simulink model "files_continuous_write_test"  (R2022a)
settings: Solver=FixedStepDiscrete  StartTime=0.0  StopTime=inf  FixedStep=0.001  MaxStep=0.001  RelTol=1e-3
undefined symbols (not defined in the file): CR, LF
libraries: dspstat3 x4, simulink x3, instrumentlib x2, matrix_library x1, slrealtimeutilitieslib x1, commcrc2 x1
settings Model: SimulationMode=accelerator  Creator=DeveloperY  LastModifiedBy=DeveloperY
settings SolverCC: AllowMultiTaskInputOutput=on  ConcurrentTasks=on

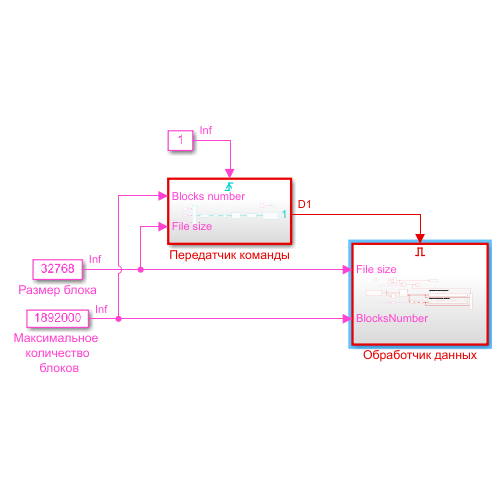
[thumbnail: Simulink's stored preview of the top-level diagram]
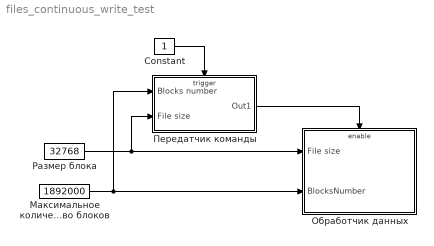
== system files_continuous_write_test ==
  Constant : Constant
  Максимальное количество блоков : Constant  Value=1892000  OutDataTypeStr=uint32
  Обработчик данных : Subsystem  TreatAsAtomicUnit=on
  Передатчик команды : Subsystem  TreatAsAtomicUnit=on
  Размер блока : Constant  Value=32768  OutDataTypeStr=uint32
  wires:
  Constant/1 -> Передатчик команды/Trigger
  Максимальное количество блоков/1 -> Передатчик команды/1(Blocks number), Обработчик данных/2(BlocksNumber)
  Размер блока/1 -> Обработчик данных/1(File size), Передатчик команды/2(File size)
  Передатчик команды/1(Out1) -> Обработчик данных/Enable

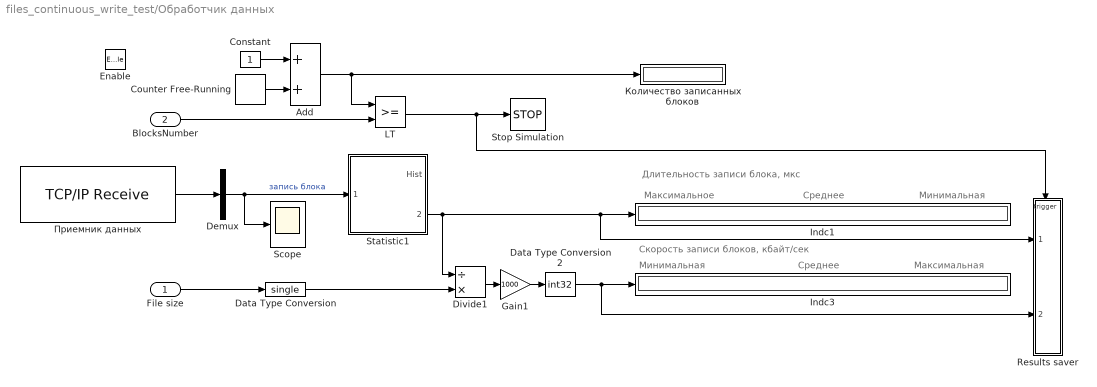
== system files_continuous_write_test/Обработчик данных ==
  note: Длительность записи блока, мкс
  note: Минимальная
  note: Среднее
  note: Максимальное
  note: Максимальная
  note: Среднее
  note: Минимальная
  note: Скорость записи блоков, кбайт/сек
  File size : Inport
  BlocksNumber : Inport  Port=2
  Enable : EnablePort
  " Indc1" : Display
  Add : Sum
  Constant : Constant
  Counter Free-Running : simulink/Sources/Counter Free-Running  NumBits=32  tsamp=-1
  Data Type Conversion : DataTypeConversion  OutDataTypeStr=single  SaturateOnIntegerOverflow=off  RndMeth=Floor
  Data Type Conversion2 : DataTypeConversion  OutDataTypeStr=int32  SaturateOnIntegerOverflow=off  RndMeth=Floor
  Demux : Demux  Outputs=1
  Divide1 : Product  Inputs=/*  OutDataTypeStr=single
  Gain1 : Gain  Gain=1000
  Indc3 : Display
  LT : RelationalOperator  OutDataTypeStr=boolean  RndMeth=Simplest  InputSameDT=off
  Results saver : Subsystem  TreatAsAtomicUnit=on
  Scope : Scope
  Statistic1 : Subsystem
  Stop Simulation : Stop
  Количество записанных блоков : Display
  Приемник данных : instrumentlib/TCP//IP Receive  Host=192.168.3.1  Port=3333  DataSize=[1]  DataType=ASCII  ASCIIFormatting=%d  Terminator=CR/LF  CustomTerminator=10  ByteOrder=big-endian  EnableBlockingMode=on  Timeout=10  SampleTime=-1  SimulateUsing=Interpreted execution
  wires:
  Demux/1 -> Scope/1, Statistic1/1(Samples)  "запись блока"
  Add/1 -> LT/1, Количество записанных блоков/1
  Statistic1/2(Duration) -> Divide1/1, " Indc1"/1, Results saver/1(Duration)
  File size/1 -> Data Type Conversion/1
  LT/1 -> Stop Simulation/1, Results saver/Trigger
  Data Type Conversion/1 -> Divide1/2
  Gain1/1 -> Data Type Conversion2/1
  Data Type Conversion2/1 -> Results saver/2(Speed), Indc3/1
  Divide1/1 -> Gain1/1
  BlocksNumber/1 -> LT/2
  Counter Free-Running/1 -> Add/2
  Constant/1 -> Add/1
  Приемник данных/1 -> Demux/1

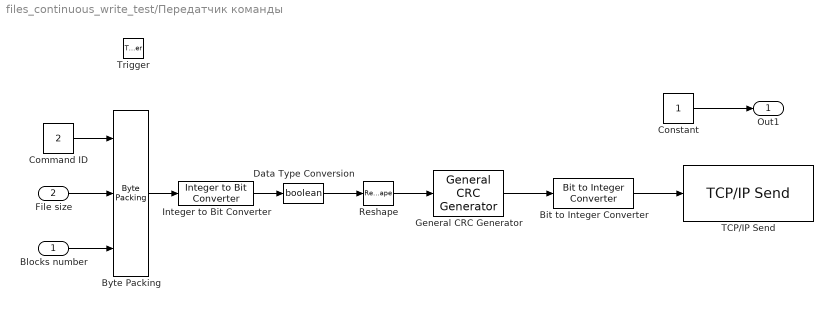
== system files_continuous_write_test/Передатчик команды ==
  Blocks number : Inport
  File size : Inport  Port=2
  Trigger : TriggerPort  VariantControl=(inherit)  InitialTriggerSignalState=zero
  Bit to Integer Converter : simulink/Logic and Bit Operations/Bit to Integer Converter  nbits=8  bitOrder=MSB first  signedOutputValues=Unsigned  outDtype=Inherit via internal rule  outDtypeSigned=Inherit via internal rule
      settings: SourceProductBaseCode=SL
  Byte Packing : slrealtimeutilitieslib/Byte Packing  MaskPackedDataType=uint8  MaskUnpackedDataTypes={'uint32','uint32','uint32' }  MaskAlignment=1
  Command ID : Constant  Value=2  OutDataTypeStr=uint32
  Constant : Constant
  Data Type Conversion : DataTypeConversion  OutDataTypeStr=boolean  SaturateOnIntegerOverflow=off  RndMeth=Floor
  General CRC Generator : commcrc2/General CRC Generator  genPoly='z^16 + z^12 + z^5 + 1'  iniStates=0  directMethod=off  reflectInputBytes=off  reflectChecksums=off  finalXOR=0  numChecksums=1
      settings: SourceProductBaseCode=CM
  Integer to Bit Converter : simulink/Logic and Bit Operations/Integer to Bit Converter  nbits=8  signedInputValues=Unsigned  bitOrder=MSB first  outDtype=Inherit via internal rule
      settings: SourceProductBaseCode=SL
  Reshape : Reshape  OutputDimensionality=Customize  OutputDimensions=[96,1]
  TCP/IP Send : instrumentlib/TCP//IP Send  Host=192.168.3.1  Port=3333  ByteOrder=big-endian  EnableBlockingMode=off  Timeout=0.1  TransferDelay=on  SimulateUsing=Interpreted execution
  Out1 : Outport
  wires:
  Command ID/1 -> Byte Packing/1
  File size/1 -> Byte Packing/2
  Blocks number/1 -> Byte Packing/3
  Integer to Bit Converter/1 -> Data Type Conversion/1
  Data Type Conversion/1 -> Reshape/1
  Reshape/1 -> General CRC Generator/1
  General CRC Generator/1 -> Bit to Integer Converter/1
  Bit to Integer Converter/1 -> TCP/IP Send/1
  Byte Packing/1 -> Integer to Bit Converter/1
  Constant/1 -> Out1/1

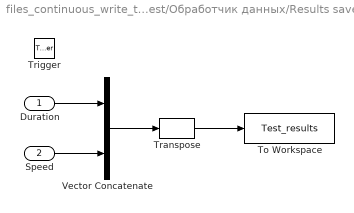
== system files_continuous_write_test/Обработчик данных/Results saver ==
  Duration : Inport
  Speed : Inport  Port=2
  Trigger : TriggerPort  VariantControl=(inherit)  InitialTriggerSignalState=zero
  To Workspace : ToWorkspace  VariableName=Test_results  SampleTime=-1
  Transpose : matrix_library/Transpose
      settings: SourceProductBaseCode=SL
  Vector Concatenate : Concatenate  Mode=Multidimensional array  ConcatenateDimension=2
  wires:
  Duration/1 -> Vector Concatenate/1
  Vector Concatenate/1 -> Transpose/1
  Transpose/1 -> To Workspace/1
  Speed/1 -> Vector Concatenate/2

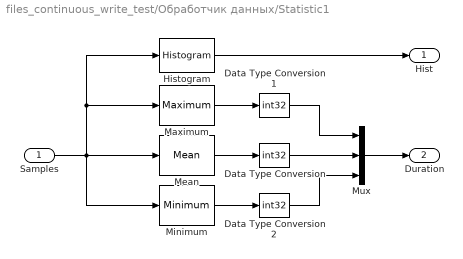
== system files_continuous_write_test/Обработчик данных/Statistic1 ==
  Samples : Inport
  Data Type Conversion : DataTypeConversion  OutDataTypeStr=int32  SaturateOnIntegerOverflow=off  RndMeth=Floor
  Data Type Conversion1 : DataTypeConversion  OutDataTypeStr=int32  SaturateOnIntegerOverflow=off  RndMeth=Floor
  Data Type Conversion2 : DataTypeConversion  OutDataTypeStr=int32  SaturateOnIntegerOverflow=off  RndMeth=Floor
  Histogram : dspstat3/Histogram  umin=0  umax=1000000  nbins=100  operateOver=Entire input  Dimension=1  normalized=off  run=on  reset=on  trigtype=None  colComp=on  roundingMode=Floor  overflowMode=off
      settings: SourceProductBaseCode=DS
  Maximum : dspstat3/Maximum  operation=maximum  fcn=Running  indexBase=One  operateOver=Specified dimension  Dimension=1  reset=None  roiEnable=off  roiType=Rectangles  roiPortion=Entire ROI  roiOutput=Individual statistics for each ROI  roiFlag=off  roundingMode=Floor  overflowMode=off  accumDataTypeStr=Inherit: Same as product output  accumLastDataTypeStr=Inherit: Same as product output
  Mean : dspstat3/Mean  run=on  reset_popup=None  directionMode=Entire input  dimension=1  roiEnable=off  roiType=Rectangles  roiPortion=Entire ROI  roiOutput=Individual statistics for each ROI  roiFlag=off  roundingMode=Floor  overflowMode=off  outputDataTypeStr=Inherit: Same as accumulator  outputMin=[]  outputMax=[]  outputLastDataTypeStr=Inherit: Same as accumulator
  Minimum : dspstat3/Minimum  operation=minimum  fcn=Running  indexBase=One  operateOver=Entire input  Dimension=1  reset=None  roiEnable=off  roiType=Rectangles  roiPortion=Entire ROI  roiOutput=Individual statistics for each ROI  roiFlag=off  roundingMode=Floor  overflowMode=off
      settings: SourceProductBaseCode=DS
  Mux : Mux  Inputs=3
  Hist : Outport
  Duration : Outport  Port=2
  wires:
  Histogram/1 -> Hist/1
  Maximum/1 -> Data Type Conversion1/1
  Minimum/1 -> Data Type Conversion2/1
  Samples/1 -> Maximum/1, Histogram/1, Minimum/1, Mean/1
  Mean/1 -> Data Type Conversion/1
  Data Type Conversion/1 -> Mux/2
  Data Type Conversion1/1 -> Mux/1
  Data Type Conversion2/1 -> Mux/3
  Mux/1 -> Duration/1
